simulink model "GFOL_linear2"  (R2020a)
settings: Solver=ode3  StartTime=0.0  StopTime=Tsim  FixedStep=T_solver  RelTol=1e-5  EnableMultiTasking=on
values from neighbouring files (symbols this model uses):
  Afdroop_n1 = [-1/tau_droop_f]    [linear_model.m]
  Ais_n1 = [0 0 ... (first row only)    [linear_model.m]
  Aisc_n1 = [0]    [linear_model.m]
  Ap_n1 = [0]    [linear_model.m]
  Apll_n1 = [0]    [linear_model.m]
  Aq_n1 = [0]    [linear_model.m]
  Arl_n1 = [-(Rc_n1+Rg_t+R_pscad)/(Lc_n1+Lg_t) -w_n1 ... (first row only)    [linear_model.m]
  Atheta_n1 = [0]    [linear_model.m]
  Au_n1 = [0]    [linear_model.m]
  Auc_n1 = [0]    [linear_model.m]
  Audroop_n1 = [-1/tau_droop_u]    [linear_model.m]
  Avcc_n1 = [0]    [linear_model.m]
  Bfdroop_n1 = [0 1]    [linear_model.m]
  Bis_n1 = [1 0 -1 0 0 0 ... (first row only)    [linear_model.m]
  Bisc_n1 = [0 0 0]    [linear_model.m]
  Bp_n1 = [1 -3/2*u_q0_n1c -3/2*u_d0_n1c -3/2*is_q0_n1c -3/2*is_d0_n1c]    [linear_model.m]
  Bpll_n1 = [1]    [linear_model.m]
  Bq_n1 = [1 +3/2*u_d0_n1c -3/2*u_q0_n1c -3/2*is_d0_n1c +3/2*is_q0_n1c]    [linear_model.m]
  Brl_n1 = [+1/(Lc_n1+Lg_t) 0 -1/(Lc_n1+Lg_t) 0 ... (first row only)    [linear_model.m]
  Btheta_n1 = [1 -1]    [linear_model.m]
  Bu_n1 = [0 0]    [linear_model.m]
  Buc_n1 = [0 0 0]    [linear_model.m]
  Budroop_n1 = [0 1]    [linear_model.m]
  Bvcc_n1 = [0 0 0]    [linear_model.m]
  Cfdroop_n1 = [-k_droop_f_n1/tau_droop_f]    [linear_model.m]
  Cis_n1 = [+ki_s_n1 0 ... (first row only)    [linear_model.m]
  Cisc_n1 = [0 ... (first row only)    [linear_model.m]
  Cp_n1 = [ki_P_n1]    [linear_model.m]
  Cpll_n1 = [-ki_pll_n1]    [linear_model.m]
  Cq_n1 = [ki_Q_n1]    [linear_model.m]
  Crl_n1 = [1 0 ... (first row only)    [linear_model.m]
  Ctheta_n1 = [1]    [linear_model.m]
  Cu_n1 = [0]    [linear_model.m]
  Cuc_n1 = [0 ... (first row only)    [linear_model.m]
  Cudroop_n1 = [-k_droop_u_n1/tau_droop_u]    [linear_model.m]
  Cvcc_n1 = [0 ... (first row only)    [linear_model.m]
  Dfdroop_n1 = [+k_droop_f_n1 0]    [linear_model.m]
  Dis_n1 = [+kp_s_n1 0 -kp_s_n1 +w_n1*Lc_n1 1 0 ... (first row only)    [linear_model.m]
  Disc_n1 = [cos(etheta0_n1) -sin(etheta0_n1) -sin(etheta0_n1)*is_q0_n1g-cos(etheta0_n1)*is_d0_n1g ... (first row only)    [linear_model.m]
  Dp_n1 = [kp_P_n1 -3/2*u_q0_n1c*kp_P_n1 -3/2*u_d0_n1c*kp_P_n1 -3/2*is_q0_n1c*kp_P_n1 -3/2*is_d0_n1c*kp_P_n1]    [linear_model.m]
  Dpll_n1 = [-kp_pll_n1]    [linear_model.m]
  Dq_n1 = [kp_Q_n1 +3/2*u_d0_n1c*kp_Q_n1 -3/2*u_q0_n1c*kp_Q_n1 -3/2*is_d0_n1c*kp_Q_n1 +3/2*is_q0_n1c*kp_Q_n1]    [linear_model.m]
  Drl_n1 = [0 0 0 0 ... (first row only)    [linear_model.m]
  Dtheta_n1 = [0 0]    [linear_model.m]
  Du_n1 = [u_q0_n1c/(sqrt(u_q0_n1c^2+u_d0_n1c^2)) u_d0_n1c/(sqrt(u_q0_n1c^2+u_d0_n1c^2))]    [linear_model.m]
  Duc_n1 = [cos(etheta0_n1) -sin(etheta0_n1) -sin(etheta0_n1)*u_q0_n1g-cos(etheta0_n1)*u_d0_n1g ... (first row only)    [linear_model.m]
  Dudroop_n1 = [+k_droop_u_n1 0]    [linear_model.m]
  Dvcc_n1 = [cos(etheta0_n1) sin(etheta0_n1) -sin(etheta0_n1)*vc_q0_n1c+cos(etheta0_n1)*vc_d0_n1c ... (first row only)    [linear_model.m]
  freq0_real_n1 = freq_real_n1(index0)    [linear_model.m]
  is_d0_n1c = is_d_real_n1c(index0)    [linear_model.m]    (also in linearization_point.m)
  is_d0_n1g = is_d_real_n1g(index0)    [linear_model.m]    (also in linearization_point.m)
  is_q0_n1c = is_q_real_n1c(index0)    [linear_model.m]    (also in linearization_point.m)
  is_q0_n1g = is_q_real_n1g(index0)    [linear_model.m]    (also in linearization_point.m)
  plots_step = 10e-6    (= 1e-05)    [param.m]
  T_solver = 10e-6    (= 1e-05)    [param.m]
  T_step = 2    [param.m]
  u_d0_n1c = u_d_real_n1c(index0)    [linear_model.m]    (also in linearization_point.m)
  u_d0_n1g = u_d_real_n1g(index0)    [linear_model.m]    (also in linearization_point.m)
  u_q0_n1c = u_q_real_n1c(index0)    [linear_model.m]    (also in linearization_point.m)
  u_q0_n1g = u_q_real_n1g(index0)    [linear_model.m]    (also in linearization_point.m)
  vc_d0_n1c = vc_d_real_n1c(index0)    [linear_model.m]    (also in linearization_point.m)
  vc_d0_n1g = vc_d_real_n1g(index0)    [linearization_point.m]
  vc_q0_n1c = vc_q_real_n1c(index0)    [linear_model.m]    (also in linearization_point.m)
  vc_q0_n1g = vc_q_real_n1g(index0)    [linearization_point.m]
  Vpeak_g1_fnl = Vpeak_n1*0.98    [param.m]
  Vpeak_n1 = Un_n1/sqrt(3)*sqrt(2)    [param.m]
  Vpeak_q1_init = Vpeak_n1*1    [param.m]
libraries: cstblocks x1
settings Model: SimulationMode=accelerator  Creator=Agustí  LastModifiedBy=Saman
settings SolverCC: ZeroCrossAlgorithm=Adaptive
settings DataIOCC: LimitDataPoints=on  SaveFormat=Array  SignalLoggingSaveFormat=ModelDataLogs  ReturnWorkspaceOutputs=off
settings OptimizationCC: BlockReduction=off  BufferReuse=off  ExpressionDepthLimit=2147483647  LifeSpan=inf
settings DebuggingCC: AlgebraicLoopMsg=none  UnderspecifiedInitializationDetection=Classic  MergeDetectMultiDrivingBlocksExec=none  FcnCallInpInsideContextMsg=warning  UnconnectedInputMsg=none  UnconnectedOutputMsg=none  UnconnectedLineMsg=none  AllowSymbolicDim=off  StateNameClashWarn=warning  SFUnexpectedBacktrackingDiag=warning  SFNoUnconditionalDefaultTransitionDiag=warning  SFExecutionAtInitializationDiag=none  ArithmeticOperatorsInVariantConditions=warning
settings HardwareCC: ProdBitPerPointer=32  ProdBitPerSizeT=32  ProdBitPerPtrDiffT=32  ProdLargestAtomicFloat=None  ProdIntDivRoundTo=Undefined  ProdEndianess=Unspecified  ProdWordSize=32  ProdHWDeviceType=32-bit Generic
settings ModelReferenceCC: PropagateSignalLabelsOutOfModel=off
settings SFSimCC: SimUseLocalCustomCode=off  CustomCodeUndefinedFunction=UseInterfaceOnly
settings RTWCC: RTWUseLocalCustomCode=off
settings CodeAppCC: StateflowObjectComments=on
settings GRTTargetCC: TargetLangStandard=C89/C90 (ANSI)
settings ConfigComp: CovMetricSettings=dw  CovHtmlReporting=on  CovSaveCumulativeToWorkspaceVar=on  CovSaveSingleToWorkspaceVar=on  CovExternalEMLEnable=off  CovSFcnEnable=off
settings SimscapeCC: SimscapeNormalizeSystem=off
settings ConfigurationSet: Description=SimMechanics 2G

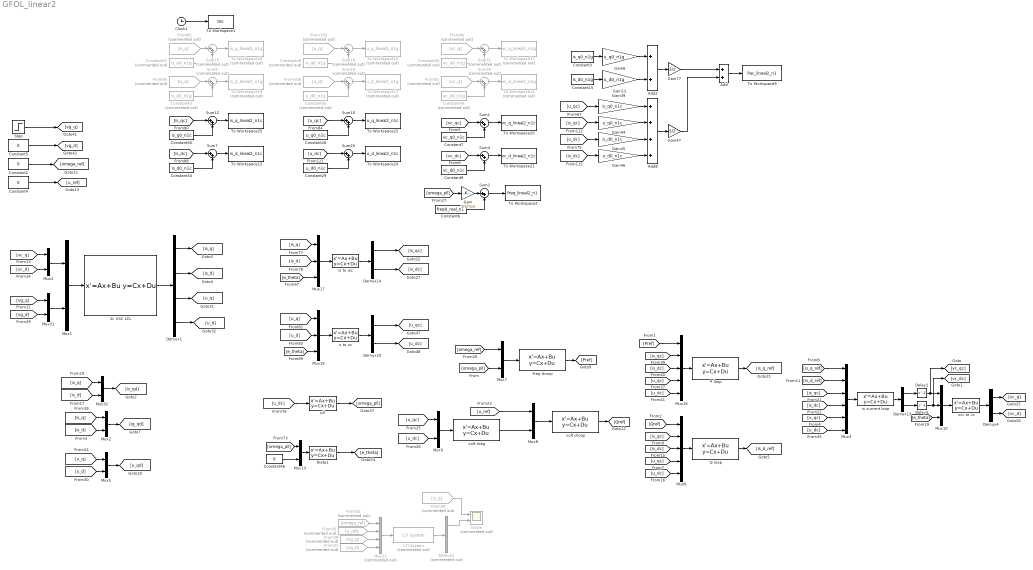
== system GFOL_linear2 ==
  2L VSC LCL : StateSpace  A=Arl_n1  B=Brl_n1  C=Crl_n1  D=Drl_n1  InitialCondition=[0 0]
  Add : Sum
  Add2 : Sum
  Add8 : Sum  Inputs=++++
  Clock1 : Clock
  Constant15 : Constant  Value=is_d0_n1g
  Constant{2,4..5,46} (4 alike) : Constant  Value=0
  Constant28 : Constant  Value=u_q0_n1c
  Constant29 : Constant  Value=u_d0_n1c
  Constant3 : Constant  Value=is_q0_n1g
  Constant30 : Constant  Value=is_q0_n1c
  Constant34 : Constant  Value=is_d0_n1c
  Constant42 : Constant  Commented=on  Value=is_q0_n1g
  Constant43 : Constant  Commented=on  Value=is_d0_n1g
  Constant44 : Constant  Commented=on  Value=vc_q0_n1g
  Constant45 : Constant  Commented=on  Value=vc_d0_n1g
  Constant49 : Constant  Commented=on  Value=u_q0_n1g
  Constant50 : Constant  Commented=on  Value=u_d0_n1g
  Constant6 : Constant  Value=freq0_real_n1
  Constant7 : Constant  Value=vc_q0_n1c
  Constant9 : Constant  Value=vc_d0_n1c
  Delay2 : Delay  DelayLength=1  InitialCondition=0  SampleTime=T_solver
  Delay5 : Delay  DelayLength=1  InitialCondition=0  SampleTime=T_solver
  Demux1 : Demux
  Demux{4,10,13..14} (4 alike) : Demux  Outputs=2
  Demux2 : Demux  Commented=on  Outputs=2
  From105 : From  Commented=on  GotoTag=u_q
  From106 : From  Commented=on  GotoTag=u_d
  From28 : From  Commented=on  GotoTag=vg_q
  From31 : From  Commented=on  GotoTag=vg_d
  From32 : From  Commented=on  GotoTag=omega_ref
  From33 : From  Commented=on  GotoTag=u_ref
  From34 : From  Commented=on  GotoTag=is_q
  From80 : From  Commented=on  GotoTag=vc_q
  From81 : From  Commented=on  GotoTag=vc_d
  From85 : From  Commented=on  GotoTag=is_q
  From86 : From  Commented=on  GotoTag=is_d
  Gain : Gain  Gain=1/(2*pi)
  Gain12 : Gain  Gain=u_d0_n1g
  Gain39 : Gain  Gain=is_q0_n1c
  Gain44 : Gain  Gain=u_q0_n1c
  Gain45 : Gain  Gain=is_d0_n1c
  Gain46 : Gain  Gain=u_d0_n1c
  Gain47 : Gain  Gain=3/2
  Gain6 : Gain  Gain=u_q0_n1g
  Gain77 : Gain  Gain=3/2
  LTI System : cstblocks/LTI System  Commented=on  sys=ss_sys  IC=zeros(1,10)
  Mux{1..2,4..5,7..9,13,31..32} (10 alike) : Mux  Inputs=2
  Mux10 : Mux  Inputs=3
  Mux11 : Mux  Commented=on
  Mux16 : Mux  Inputs=5
  Mux17 : Mux  Inputs=3
  Mux19 : Mux  Inputs=3
  Mux3 : Mux  Inputs=6
  Mux6 : Mux  Inputs=5
  P loop : StateSpace  A=Ap_n1  B=Bp_n1  C=Cp_n1  D=Dp_n1  InitialCondition=[0]
  Q loop : StateSpace  A=Aq_n1  B=Bq_n1  C=Cq_n1  D=Dq_n1  InitialCondition=[0]
  Scope : Scope  Commented=on  NumInputPorts=2
  Step : Step  Time=T_step  Before=Vpeak_q1_init-Vpeak_n1  After=Vpeak_g1_fnl-Vpeak_n1  SampleTime=0
  Sum{1..2,4,7,10,12,20} (7 alike) : Sum  Inputs=|++
  Sum{9,14,19,25,30..31} (6 alike) : Sum  Commented=on  Inputs=|++
  To Workspace1 : ToWorkspace  VariableName=tlin  SampleTime=plots_step
  To Workspace13 : ToWorkspace  Commented=on  VariableName=vc_q_lineal2_n1g  SampleTime=plots_step
  To Workspace14 : ToWorkspace  Commented=on  VariableName=vc_d_lineal2_n1g  SampleTime=plots_step
  To Workspace15 : ToWorkspace  VariableName=is_d_lineal2_n1c  SampleTime=plots_step
  To Workspace16 : ToWorkspace  Commented=on  VariableName=u_q_lineal2_n1g  SampleTime=plots_step
  To Workspace17 : ToWorkspace  Commented=on  VariableName=u_d_lineal2_n1g  SampleTime=plots_step
  To Workspace18 : ToWorkspace  Commented=on  VariableName=is_q_lineal2_n1g  SampleTime=plots_step
  To Workspace19 : ToWorkspace  Commented=on  VariableName=is_d_lineal2_n1g  SampleTime=plots_step
  To Workspace2 : ToWorkspace  VariableName=freq_lineal2_n1  SampleTime=plots_step
  To Workspace20 : ToWorkspace  VariableName=vc_q_lineal2_n1c  SampleTime=plots_step
  To Workspace21 : ToWorkspace  VariableName=vc_d_lineal2_n1c  SampleTime=plots_step
  To Workspace22 : ToWorkspace  VariableName=u_q_lineal2_n1c  SampleTime=plots_step
  To Workspace24 : ToWorkspace  VariableName=u_d_lineal2_n1c  SampleTime=plots_step
  To Workspace25 : ToWorkspace  VariableName=is_q_lineal2_n1c  SampleTime=plots_step
  To Workspace9 : ToWorkspace  VariableName=Pac_lineal2_n1  SampleTime=plots_step
  freq droop : StateSpace  A=Afdroop_n1  B=Bfdroop_n1  C=Cfdroop_n1  D=Dfdroop_n1  InitialCondition=[0]
  is current loop : StateSpace  A=Ais_n1  B=Bis_n1  C=Cis_n1  D=Dis_n1  InitialCondition=[0 0]
  is to isc : StateSpace  A=Aisc_n1  B=Bisc_n1  C=Cisc_n1  D=Disc_n1  InitialCondition=[0]
  pll : StateSpace  A=Apll_n1  B=Bpll_n1  C=Cpll_n1  D=Dpll_n1  InitialCondition=[0]
  theta1 : StateSpace  A=Atheta_n1  B=Btheta_n1  C=Ctheta_n1  D=Dtheta_n1  InitialCondition=[0]
  u to uc : StateSpace  A=Auc_n1  B=Buc_n1  C=Cuc_n1  D=Duc_n1  InitialCondition=[0]
  vcc to vc : StateSpace  A=Avcc_n1  B=Bvcc_n1  C=Cvcc_n1  D=Dvcc_n1  InitialCondition=[0]
  volt droop : StateSpace  A=Audroop_n1  B=Budroop_n1  C=Cudroop_n1  D=Dudroop_n1  InitialCondition=[0]
  volt mag : StateSpace  A=Au_n1  B=Bu_n1  C=Cu_n1  D=Du_n1  InitialCondition=[0]
  wires:
  Clock1/1 -> To Workspace1/1
  Constant29/1 -> Sum20/2
  [e_theta] -> Mux17/3
  Sum7/1 -> To Workspace15/1
  [e_theta] -> Mux19/3
  Demux10/2 -> [u_dc]
  Sum14/1 -> To Workspace16/1
  [is_dc] -> Gain46/1
  Gain39/1 -> Add8/1
  Sum31/1 -> To Workspace13/1
  Constant42/1 -> Sum25/2
  Sum30/1 -> To Workspace14/1
  u to uc/1 -> Demux10/1
  [u_qc] -> Gain39/1
  Gain44/1 -> Add8/2
  Sum19/1 -> To Workspace17/1
  Constant43/1 -> Sum9/2
  is to isc/1 -> Demux14/1
  [u_qc] -> Mux3/5
  Demux4/1 -> [vc_q]
  Constant46/1 -> Mux13/2
  [is_qc] -> Gain44/1
  [u_dc] -> Gain45/1
  Sum9/1 -> To Workspace19/1
  From85/1 -> Sum25/1
  Gain46/1 -> Add8/4
  [u_dc] -> Sum20/1
  vcc to vc/1 -> Demux4/1
  From106/1 -> Sum19/1
  [u_dc] -> Mux16/5
  Constant34/1 -> Sum7/2
  [is_d_ref] -> Mux3/2
  Demux14/1 -> [is_qc]
  Q loop/1 -> [is_d_ref]
  [u_q] -> Mux5/1
  [e_theta] -> Mux10/3
  Sum1/1 -> To Workspace20/1
  [u_qc] -> Mux6/4
  [is_qc] -> Sum12/1
  [Qref] -> Mux6/1
  Add8/1 -> Gain47/1
  Constant28/1 -> Sum10/2
  Constant45/1 -> Sum30/2
  Gain45/1 -> Add8/3
  [is_q] -> Mux17/1
  Mux10/1 -> vcc to vc/1
  [is_qc] -> Mux16/2
  Gain77/1 -> Add/1
  [vc_dc] -> Sum4/1
  [u_dc] -> Mux6/5
  From105/1 -> Sum14/1
  Sum10/1 -> To Workspace22/1
  [u_qc] -> Mux16/4
  Mux6/1 -> Q loop/1
  Constant44/1 -> Sum31/2
  Mux31/1 -> Mux1/2
  Demux14/2 -> [is_dc]
  Demux10/1 -> [u_qc]
  Add/1 -> To Workspace9/1
  From80/1 -> Sum31/1
  [u_d] -> Mux5/2
  Mux17/1 -> is to isc/1
  Constant15/1 -> Gain12/1
  Sum25/1 -> To Workspace18/1
  Gain12/1 -> Add2/2
  theta1/1 -> [e_theta]
  Constant9/1 -> Sum4/2
  [is_qc] -> Mux6/2
  Gain6/1 -> Add2/1
  [omega_pll] -> Mux13/1
  [is_dc] -> Mux16/3
  Gain47/1 -> Add/2
  [vc_qc] -> Sum1/1
  [is_q] -> Mux2/1
  From86/1 -> Sum9/1
  Constant3/1 -> Gain6/1
  [u_d] -> Mux19/2
  Step/1 -> [vg_q]
  [is_d] -> Mux17/2
  Constant7/1 -> Sum1/2
  pll/1 -> [omega_pll]
  Mux13/1 -> theta1/1
  [is_q] -> Mux32/1
  Sum4/1 -> To Workspace21/1
  Mux32/1 -> [is_qd]
  [Pref] -> Mux16/1
  [is_d] -> Mux32/2
  [vg_d] -> Mux31/2
  Mux4/1 -> Mux1/1
  Demux1/1 -> [is_q]
  Mux2/1 -> [ig_qd]
  From81/1 -> Sum30/1
  Mux16/1 -> P loop/1
  Constant49/1 -> Sum14/2
  Demux13/2 -> Delay5/1
  Add2/1 -> Gain77/1
  Mux1/1 -> 2L VSC LCL/1
  Mux5/1 -> [u_qd]
  Constant50/1 -> Sum19/2
  [vc_d] -> Mux4/2
  Mux19/1 -> u to uc/1
  Demux1/2 -> [is_d]
  [vc_q] -> Mux4/1
  [is_d] -> Mux2/2
  [is_dc] -> Mux6/3
  Demux4/2 -> [vc_d]
  [vg_q] -> Mux31/1
  Constant30/1 -> Sum12/2
  Demux1/4 -> [u_d]
  [u_dc] -> pll/1
  2L VSC LCL/1 -> Demux1/1
  Sum12/1 -> To Workspace25/1
  is current loop/1 -> Demux13/1
  P loop/1 -> [is_q_ref]
  [u_qc] -> Sum10/1
  [is_dc] -> Sum7/1
  [is_dc] -> Mux3/4
  Sum20/1 -> To Workspace24/1
  Demux13/1 -> Delay2/1
  Constant5/1 -> [vg_d]
  [is_q_ref] -> Mux3/1
  [is_qc] -> Mux3/3
  Mux3/1 -> is current loop/1
  [u_q] -> Mux19/1
  Demux1/3 -> [u_q]
  [u_dc] -> Mux3/6
  Delay5/1 -> [vc_dc], Mux10/2
  Delay2/1 -> [vc_qc], Mux10/1
  Mux7/1 -> freq droop/1
  [omega_pll] -> Mux7/2
  [omega_ref] -> Mux7/1
  Constant2/1 -> [omega_ref]
  Mux8/1 -> volt droop/1
  Mux9/1 -> volt mag/1
  volt mag/1 -> Mux8/2
  [u_ref] -> Mux8/1
  Constant4/1 -> [u_ref]
  [u_qc] -> Mux9/1
  [u_dc] -> Mux9/2
  [omega_pll] -> Gain/1
  Constant6/1 -> Sum2/2
  Gain/1 -> Sum2/1
  Sum2/1 -> To Workspace2/1
  freq droop/1 -> [Pref]
  volt droop/1 -> [Qref]
  Mux11/1 -> LTI System/1
  LTI System/1 -> Demux2/1
  From28/1 -> Mux11/3
  From31/1 -> Mux11/4
  From32/1 -> Mux11/1
  From33/1 -> Mux11/2
  From34/1 -> Scope/1
  Demux2/1 -> Scope/2
